simulink model "Part5"  (R2024b)
settings: Solver=VariableStepAuto  StartTime=0.0  StopTime=5  MaxStep=0.001  RelTol=1e-3
values from neighbouring files (symbols this model uses):
  A = [0, 1; 0, -1/Tm]    [DesignPart567.m]    (also in DesignPart8.m; DesignPart9Sine.m; DesignPart9Step.m = [0, 1; 0, a22]; Init.m = [0, 1;0, -1/Tm])
  B = [0, km/(gbox.N*Tm)]'    [DesignPart567.m]    (also in DesignPart8.m; DesignPart9Sine.m; DesignPart9Step.m = [0, b2]'; Init.m = [0; drv.dcgain*mot.Kt/(gbox.N1*mot.Req*Jeq)])
  C = [1, 0]    [DesignPart567.m]    (also in DesignPart8.m; DesignPart9Sine.m; DesignPart9Step.m; Init.m)
  Cr = [90, 0]    [DesignPart567.m]    (also in DesignPart8.m = 90)
  delta_est = 1/sqrt(2)    [DesignPart9Step.m]    (also in Init.m)
  K = real(K)    [DesignPart567.m]    (also in DesignPart8.m; DesignPart9Sine.m; DesignPart9Step.m = place(  A,   B, CtrlPoles); Init.m = acker(A,B,poles))
  W0 = 1/Tr    (= 10)    [DesignPart567.m]    (also in DesignPart9Sine.m = 2*pi/Tr)
  wc = 2*pi*50    (= 314.159265359)    [DesignPart9Step.m]    (also in Init.m; State_space_1324.m)
undefined symbols (not defined in the file or in its folder): drv, sens
libraries: simulink_extras x3
settings Model: Creator=Banaan  LastModifiedBy=Banaan

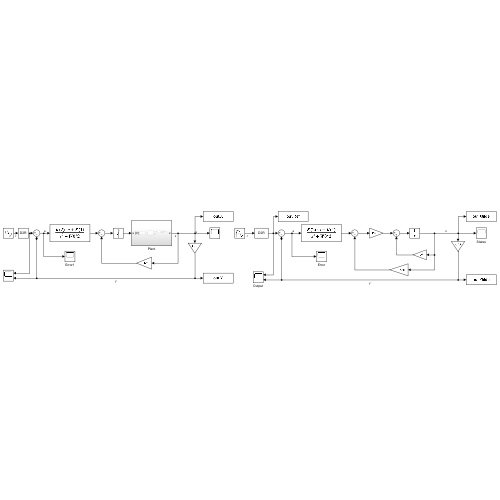
[thumbnail: Simulink's stored preview of the top-level diagram]
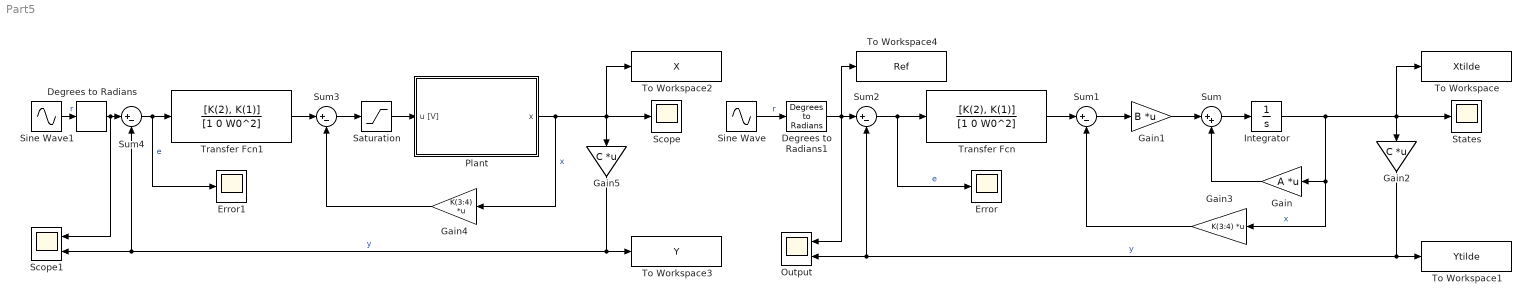
== system Part5 ==
  Degrees to Radians : simulink_extras/Transformations/Degrees to Radians
  Degrees to Radians1 : simulink_extras/Transformations/Degrees to Radians
  Error : Scope
  Error1 : Scope
  Gain : Gain  Gain=A  Multiplication=Matrix(K*u)
  Gain1 : Gain  Gain=B  Multiplication=Matrix(K*u)
  Gain2 : Gain  Gain=C  Multiplication=Matrix(K*u)
  Gain3 : Gain  Gain=K(3:4)  Multiplication=Matrix(K*u)
  Gain4 : Gain  Gain=K(3:4)  Multiplication=Matrix(K*u)
  Gain5 : Gain  Gain=C  Multiplication=Matrix(K*u)
  Integrator : Integrator  InitialCondition=rand(2, 1)
  Output : Scope  NumInputPorts=2
  Plant : Subsystem
  Saturation : Saturate  UpperLimit=10  LowerLimit=-10
  Scope : Scope
  Scope1 : Scope  NumInputPorts=2
  Sine Wave : Sin  Amplitude=Cr(1)  Frequency=W0  SampleTime=0
  Sine Wave1 : Sin  Amplitude=Cr(1)  Frequency=W0  SampleTime=0
  States : Scope
  Sum : Sum  Inputs=|++
  Sum{1..4} (4 alike) : Sum  Inputs=|+-
  To Workspace : ToWorkspace  VariableName=Xtilde  SaveFormat=Timeseries  SampleTime=-1
  To Workspace1 : ToWorkspace  VariableName=Ytilde  SaveFormat=Timeseries  SampleTime=-1
  To Workspace2 : ToWorkspace  VariableName=X  SaveFormat=Timeseries  SampleTime=-1
  To Workspace3 : ToWorkspace  VariableName=Y  SaveFormat=Timeseries  SampleTime=-1
  To Workspace4 : ToWorkspace  VariableName=Ref  SaveFormat=Timeseries  SampleTime=-1
  Transfer Fcn : TransferFcn  Numerator=[K(2), K(1)]  Denominator=[1 0 W0^2]
  Transfer Fcn1 : TransferFcn  Numerator=[K(2), K(1)]  Denominator=[1 0 W0^2]
  wires:
  Integrator/1 -> Gain/1, Gain3/1, To Workspace/1, Gain2/1, States/1  "x"
  Gain/1 -> Sum/2
  Sum/1 -> Integrator/1
  Gain1/1 -> Sum/1
  Sum1/1 -> Gain1/1
  Gain2/1 -> To Workspace1/1, Sum2/2, Output/2  "y"
  Gain3/1 -> Sum1/2
  Transfer Fcn/1 -> Sum1/1
  Sum2/1 -> Error/1, Transfer Fcn/1  "e"
  Sum3/1 -> Saturation/1
  Gain4/1 -> Sum3/2
  Sum4/1 -> Transfer Fcn1/1, Error1/1  "e"
  Gain5/1 -> To Workspace3/1, Scope1/2, Sum4/2  "y"
  Transfer Fcn1/1 -> Sum3/1
  Plant/1(x) -> To Workspace2/1, Gain5/1, Scope/1, Gain4/1  "x"
  Saturation/1 -> Plant/1(u [V])
  Sine Wave1/1 -> Degrees to Radians/1  "r"
  Degrees to Radians/1 -> Scope1/1, Sum4/1
  Sine Wave/1 -> Degrees to Radians1/1  "r"
  Degrees to Radians1/1 -> Output/1, To Workspace4/1, Sum2/1

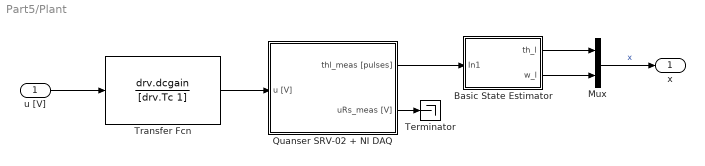
== system Part5/Plant ==
  u [V] : Inport
  Basic State Estimator : Subsystem
  Mux : Mux  Inputs=2
  Quanser SRV-02 + NI DAQ : Subsystem  mask(Quanser SRV-02 (with inertial load) + NI DAQ){Ts=0.001, fricType=Coulomb + viscous}
      mask prompts: Ts "NI DAQ Sample Time:"; fricType "Friction model"
      mask help: Quanser SRV-02 (with inertial load) + NI DAQ model.
      mask init:
      | %%  Sensors data
      | 
      | %   shunt resistor
      | sens.curr.Rs = 0.5;                         %   resistance [Ohm]   
      | sens.curr.uRs_std = 0.01;                   %   voltage noise standard dev [V]                           
      | sens.curr.uRs_var = sens.curr.uRs_std^2;	%   voltage noise variance [V^2]
      | 
      | %   Hewlett-Packard HEDS-5540#A06 optical encoder
      | sens.enc.ppr = 500*4;                       %   pulses per rotation
      | sens.enc.pulse2deg = 360/sens.enc.ppr;      %   [pulses] -> [deg]
      | sens.enc.pulse2rad = 2*pi/sens.enc.ppr;     %   [pulses] -> [rad]
      | sens.enc.deg2pulse = sens.enc.ppr/360;      %   [deg] -> [pulses]
      | sens.enc.rad2pulse = sens.enc.ppr/2/pi;     %   [rad] -> [pulses]
      | 
      | 
      | %%  Data acquisition board (daq) data
      | 
      | %   NI PCI-6221 DAC data
      | daq.dac.bits = 16;                                  %   resolution (bits)
      | daq.dac.fs   = 10;                                  %   full scale 
      | daq.dac.q    = 2*daq.dac.fs/(2^daq.dac.bits-1);     %	quantization
      | 
      | %   NI PCI-6221 ADC data
      | daq.adc.bits = 16;                                  %   resolution (bits)
      | daq.adc.fs   = 10;                                  %   full scale (as set in SLDRT Analog Input block)
      | daq.adc.q    = 2*daq.adc.fs/(2^daq.adc.bits-1);     %   quantization
      mask Help:
      | Riccardo Antonello (antonello@dei.unipd.it)
      | 
      | April 24, 2020
      | 
      | Dept. of Information Engineering, University of Padova
      mask TypeOptions fricType: Coulomb + viscous | Karnopp
  Terminator : Terminator
  Transfer Fcn : TransferFcn  Numerator=drv.dcgain  Denominator=[drv.Tc 1]
  x : Outport
  wires:
  u [V]/1 -> Transfer Fcn/1
  Quanser SRV-02 + NI DAQ/1(thl_meas [pulses]) -> Basic State Estimator/1(In1)
  Mux/1 -> x/1  "x"
  Quanser SRV-02 + NI DAQ/2(uRs_meas [V]) -> Terminator/1
  Transfer Fcn/1 -> Quanser SRV-02 + NI DAQ/1(u [V])
  Basic State Estimator/1(th_l) -> Mux/1
  Basic State Estimator/2(w_l) -> Mux/2

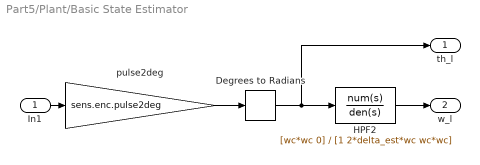
== system Part5/Plant/Basic State Estimator ==
  In1 : Inport
  Degrees to Radians : simulink_extras/Transformations/Degrees to Radians
  HPF2 : TransferFcn  Numerator=[wc*wc 0]  Denominator=[1 2*delta_est*wc wc*wc]
  pulse2deg : Gain  Gain=sens.enc.pulse2deg
  th_l : Outport
  w_l : Outport  Port=2
  wires:
  pulse2deg/1 -> Degrees to Radians/1
  In1/1 -> pulse2deg/1
  HPF2/1 -> w_l/1
  Degrees to Radians/1 -> th_l/1, HPF2/1

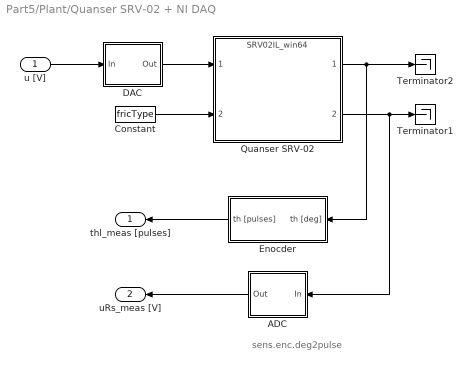
== system Part5/Plant/Quanser SRV-02 + NI DAQ ==
  note: sens.enc.deg2pulse
  u [V] : Inport
  ADC : Subsystem
  Constant : Constant  Value=fricType
  DAC : Subsystem
  Enocder : Subsystem
  Quanser SRV-02 : ModelReference  ModelNameDialog=SRV02IL_win64.slxp  ModelReferenceVersion=1.44  CopyOfModelProtected=on
  Terminator1 : Terminator
  Terminator2 : Terminator
  thl_meas [pulses] : Outport
  uRs_meas [V] : Outport  Port=2
  wires:
  Enocder/1(th [pulses]) -> thl_meas [pulses]/1
  ADC/1(Out) -> uRs_meas [V]/1
  DAC/1(Out) -> Quanser SRV-02/1
  Quanser SRV-02/2 -> ADC/1(In), Terminator1/1
  u [V]/1 -> DAC/1(In)
  Quanser SRV-02/1 -> Enocder/1(th [deg]), Terminator2/1
  Constant/1 -> Quanser SRV-02/2

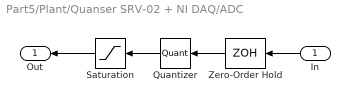
== system Part5/Plant/Quanser SRV-02 + NI DAQ/ADC ==
  In : Inport
  Quantizer : Quantizer  QuantizationInterval=daq.adc.q
  Saturation : Saturate  UpperLimit=daq.adc.fs  LowerLimit=-daq.adc.fs
  Zero-Order Hold : ZeroOrderHold  SampleTime=Ts
  Out : Outport
  wires:
  Saturation/1 -> Out/1
  In/1 -> Zero-Order Hold/1
  Quantizer/1 -> Saturation/1
  Zero-Order Hold/1 -> Quantizer/1

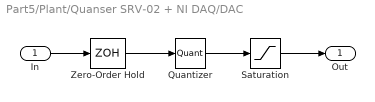
== system Part5/Plant/Quanser SRV-02 + NI DAQ/DAC ==
  In : Inport
  Quantizer : Quantizer  QuantizationInterval=daq.dac.q
  Saturation : Saturate  UpperLimit=daq.dac.fs  LowerLimit=-daq.dac.fs
  Zero-Order Hold : ZeroOrderHold  SampleTime=Ts
  Out : Outport
  wires:
  Quantizer/1 -> Saturation/1
  In/1 -> Zero-Order Hold/1
  Zero-Order Hold/1 -> Quantizer/1
  Saturation/1 -> Out/1

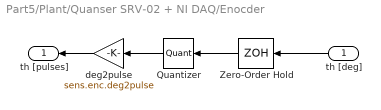
== system Part5/Plant/Quanser SRV-02 + NI DAQ/Enocder ==
  th [deg] : Inport
  Quantizer : Quantizer  QuantizationInterval=sens.enc.pulse2deg
  Zero-Order Hold : ZeroOrderHold  SampleTime=Ts
  deg2pulse : Gain  Gain=sens.enc.deg2pulse
  th [pulses] : Outport
  wires:
  Quantizer/1 -> deg2pulse/1
  th [deg]/1 -> Zero-Order Hold/1
  Zero-Order Hold/1 -> Quantizer/1
  deg2pulse/1 -> th [pulses]/1
